simulink model "SumsModel"  (Simulink 7.5)
settings: Solver=ode45  StartTime=0.0  StopTime=10  RelTol=1e-3
undefined symbols (not defined in the file or in its folder): CauchyAttribute, IntegralAttribute, n
settings Model: Creator=alexcftrk  LastModifiedBy=knifewounded

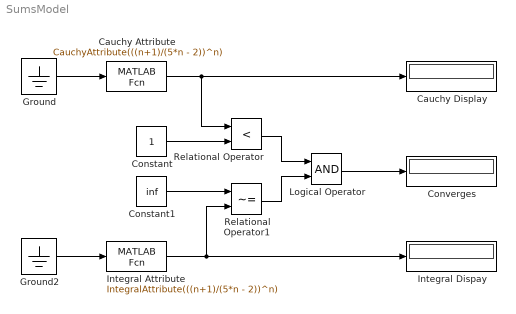
== system SumsModel ==
  Cauchy Attribute : MATLABFcn  MATLABFcn=CauchyAttribute(((n+1)/(5*n - 2))^n)
  Cauchy Display : Display
  Constant : Constant  OutDataType=fixdt(1, 16)  OutScaling=2^0
  Constant1 : Constant  Value=inf  OutDataType=fixdt(1, 16)  OutScaling=2^0
  Converges : Display
  Ground : Ground
  Ground2 : Ground
  Integral Attribute : MATLABFcn  MATLABFcn=IntegralAttribute(((n+1)/(5*n - 2))^n)
  Integral Dispay : Display
  Logical Operator : Logic  AllPortsSameDT=off  OutDataTypeMode=boolean  LogicDataType=fixdt(0, 8)  OutDataTypeStr=boolean
  Relational Operator : RelationalOperator  Operator=<  LogicOutDataTypeMode=boolean  LogicDataType=fixdt(0, 8)  OutDataTypeStr=boolean
  Relational Operator1 : RelationalOperator  Operator=~=  LogicOutDataTypeMode=boolean  LogicDataType=fixdt(0, 8)  OutDataTypeStr=boolean
  wires:
  Cauchy Attribute/1 -> Cauchy Display/1, Relational Operator/1
  Integral Attribute/1 -> Integral Dispay/1, Relational Operator1/2
  Constant/1 -> Relational Operator/2
  Logical Operator/1 -> Converges/1
  Relational Operator/1 -> Logical Operator/1
  Relational Operator1/1 -> Logical Operator/2
  Constant1/1 -> Relational Operator1/1
  Ground/1 -> Cauchy Attribute/1
  Ground2/1 -> Integral Attribute/1
